simulink model "EV_Modeling"  (R2024b)
settings: Solver=FixedStepAuto  StartTime=0.0  StopTime=3500  FixedStep=0.1  RelTol=1e-3
values from neighbouring files (symbols this model uses):
  battery_SOC_resistance = battery_SOC(:,3)    [EV_Truck.m]
  battery_SOC_SOC = battery_SOC(:,1)    [EV_Truck.m]    (also in simulink.m)
  battery_SOC_voltage = battery_SOC(:,2)    [EV_Truck.m]    (also in simulink.m)
  electric_consumption_ressistancce = electric_consumption(:,2)    [EV_Truck.m]    (also in simulink.m)
  electric_consumption_voltage = electric_consumption(:,1)    [EV_Truck.m]    (also in simulink.m)
  motor_efficiency_efficiency = table2array(motor_efficiency(2:height(motor_efficiency),2:width(motor_efficiency)))    [EV_Truck.m]    (also in simulink.m)
  motor_efficiency_RPM = table2array(motor_efficiency(2:height(motor_efficiency),1))    [EV_Truck.m]    (also in simulink.m)
  motor_efficiency_torque = transpose(motor_efficiency_torque)    [EV_Truck.m]    (also in simulink.m)
  motor_RPM_torque = table2array(motor_torque(1:14,1))    [EV_Truck.m]    (also in simulink.m)
  motor_torque_RPM = table2array(motor_torque(1:14,2))    [EV_Truck.m]    (also in simulink.m)
undefined symbols (not defined in the file or in its folder): battery_builder_rtmsupport, battery_sli_rtmsupport, DiscIntNeverNeededParam, gcbh, recurrentNet
libraries: dlutilitylib x10, dlsequencelib x10, packLibrary_lib x10, simulink x7, dlconvfclib x6, dlactivationlib x5, sharedTrackingLibrary x3, mpcadaslib x2, nesl_utility x2, fl_lib x2, slpidlib x2, simulink_extras x1
(part 8 of 9)

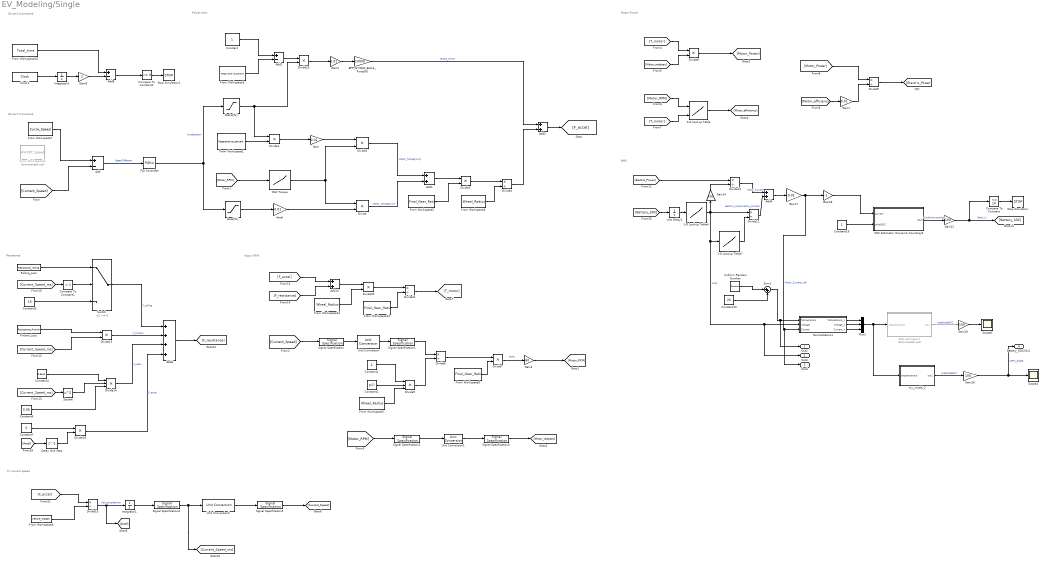
== system EV_Modeling/Single ==
  note: BMS
  note: To current speed
  note: Resistance
  note: Motor Power
  note: Power train
  note: Driver's Command
  note: RPS
  note: Motor RPM
  note: Driver's Command
  " Normalization1" : MATLAB Function  TreatAsAtomicUnit=on
  1-D Lookup Table4 : Lookup_n-D  NumberOfTableDimensions=1  BreakpointsForDimension1=battery_SOC_SOC  Table=battery_SOC_voltage  ExtrapMethod=Clip  UseLastTableValue=on  InternalRulePriority=Speed  RndMeth=Simplest
  1-D Lookup Table7 : Lookup_n-D  NumberOfTableDimensions=1  BreakpointsForDimension1=battery_SOC_SOC  Table=battery_SOC_resistance  InternalRulePriority=Speed  RndMeth=Simplest
  2-D Lookup Table : Lookup_n-D  BreakpointsForDimension1=motor_efficiency_RPM  BreakpointsForDimension2=motor_efficiency_torque  Table=motor_efficiency_efficiency  InternalRulePriority=Speed  RndMeth=Simplest
      settings: InputPortMap=u0,u1
  Accel : Gain  Gain=0.01
  Accel[%] : Saturate  UpperLimit=100  LowerLimit=0
  Add : Sum  Inputs=+-
  Add{1,3..4,10} (4 alike) : Sum
  Add2 : Sum  Inputs=+-
  Add6 : Sum  Inputs=++++
  Add8 : Sum  Inputs=+-
  BPP[%]*MAX_Brake_Force[N] : Gain  Gain=10000
  Brake[%] : Saturate  UpperLimit=0  LowerLimit=-100
  Clock1 : simulink_extras/Flip Flops/Clock  period=2
  Compare To Constant : simulink/Logic and Bit Operations/Compare To Constant  relop=<=  const=10  OutDataTypeStr=boolean
  Compare To Constant1 : simulink/Logic and Bit Operations/Compare To Constant  relop=>  const=1  OutDataTypeStr=boolean
  Compare To Constant2 : simulink/Logic and Bit Operations/Compare To Constant  relop=<=  const=0  OutDataTypeStr=boolean
  Constant : Constant
  Constant1 : Constant  Value=2
  Constant13 : Constant  Value=25
  Constant16 : Constant
  Constant2 : Constant  Value=pi()
  Constant3 : Constant  Value=10
  Constant4 : Constant  Value=0.6441
  Constant6 : Constant  Value=5.06
  Constant7 : Constant  Value=5
  Delay One Step : Delay  DelayLength=1
  Divide{,1..3,7..8,13,16,19..20} (10 alike) : Product  Inputs=**
  Divide{4,6,9,11..12,15,21} (7 alike) : Product  Inputs=*/
  Divide14 : Product  Inputs=***
  Divide5 : Product  Inputs=***
  Friction_Loss : FromWorkspace  VariableName=Resistance_friction
  From Workspace1 : FromWorkspace  VariableName=Regenerative_percent
  From Workspace10 : FromWorkspace  VariableName=Total_time
  From Workspace11 : FromWorkspace  Commented=on  VariableName=HWFET_Speed
  From Workspace12 : FromWorkspace  VariableName=Final_Gear_Ratio
  From Workspace13 : FromWorkspace  VariableName=Wheel_Radius
  From Workspace2 : FromWorkspace  VariableName=Final_Gear_Ratio
  From Workspace3 : FromWorkspace  VariableName=Regenerative_percent
  From Workspace4 : FromWorkspace  VariableName=Wheel_Radius
  From Workspace5 : FromWorkspace  VariableName=Wheel_Radius
  From Workspace6 : FromWorkspace  VariableName=Final_Gear_Ratio
  From Workspace7 : FromWorkspace  VariableName=Cycle_Speed
  From Workspace9 : FromWorkspace  VariableName=Vehicle_Weight
  Gain{,1,7,17} (4 alike) : Gain  Gain=0.01
  Gain{12,14,16,19} (4 alike) : Gain  Gain=100
  Gain18 : Gain  Gain=-1
  Gain2 : Gain  Gain=60
  Gain8 : Gain  Gain=2
  Integrator1 : Integrator
  Integrator3 : Integrator
  MAX Torque : Lookup_n-D  NumberOfTableDimensions=1  BreakpointsForDimension1=motor_RPM_torque  Table=motor_torque_RPM  InternalRulePriority=Speed  RndMeth=Simplest
  Mux2 : Mux  Inputs=3
  PID Controller : slpidlib/PID Controller  Controller=PID  Form=Parallel  TimeDomain=Continuous-time  UseExternalTs=off  SampleTime=-1  IntegratorMethod=Forward Euler  FilterMethod=Forward Euler  ControllerParametersSource=internal  P=100  I=0.01  UseKiTs=off  D=0.0001  UseExternalDerivativeSource=off  N=10  UseFilter=on  TunerSelectOption=Transfer Function Based (PID Tuner App)  InitialConditionSource=internal  InitialConditionForIntegrator=0  InitialConditionForFilter=0  DifferentiatorICPrevScaledInput=0  ExternalReset=none  TrackingMode=off  Kt=1  LimitOutput=off  SatLimitsSource=internal  UpperSaturationLimit=inf  LowerSaturationLimit=-inf  LinearizeAsGain=on  AntiWindupMode=none  Kb=1  LimitIntegrator=off  UpperIntegratorSaturationLimit=inf  LowerIntegratorSaturationLimit=-inf  POutMin=[]  POutMax=[]  IOutMin=[]  IOutMax=[]  DOutMin=[]  DOutMax=[]  NOutMin=[]  NOutMax=[]  SumOutMin=[]  SumOutMax=[]  SaturationOutMin=[]  SaturationOutMax=[]  PParamMin=[]  PParamMax=[]  IParamMin=[]  IParamMax=[]  DParamMin=[]  DParamMax=[]  NParamMin=[]  NParamMax=[]  KbParamMin=[]  KbParamMax=[]  KtParamMin=[]  KtParamMax=[]  KbOutMin=[]  KbOutMax=[]  KtOutMin=[]  KtOutMax=[]  IntegratorOutMin=[]  IntegratorOutMax=[]  FilterOutMin=[]  FilterOutMax=[]  SumI1OutMin=[]  SumI1OutMax=[]  SumI2OutMin=[]  SumI2OutMax=[]  SumI3OutMin=[]  SumI3OutMax=[]  SumI4OutMin=[]  SumI4OutMax=[]  SumDOutMin=[]  SumDOutMax=[]  DifferentiatorOutMin=[]  DifferentiatorOutMax=[]  FilterDiffOutCoefMin=[]  FilterDiffOutCoefMax=[]  ReciprocalOutMin=[]  ReciprocalOutMax=[]  SumDenOutMin=[]  SumDenOutMax=[]  SumNumOutMin=[]  SumNumOutMax=[]  DivideOutMin=[]  DivideOutMax=[]  UdiffTsProdOutMin=[]  UdiffTsProdOutMax=[]  NTsProdOutMin=[]  NTsProdOutMax=[]  UintegralTsProdOutMin=[]  UintegralTsProdOutMax=[]  UngainTsProdOutMin=[]  UngainTsProdOutMax=[]  ClampingZeroOutDataTypeStr=Inherit: Inherit via back propagation  ClampingZeroOutMin=[]  ClampingZeroOutMax=[]  FilterDenConstantOutDataTypeStr=Inherit: Inherit via back propagation  FilterDenConstantOutMin=[]  FilterDenConstantOutMax=[]  PCopyOutDataTypeStr=Inherit: Inherit via back propagation  PCopyOutMin=[]  PCopyOutMax=[]  NCopyOutDataTypeStr=Inherit: Inherit via back propagation  NCopyOutMin=[]  NCopyOutMax=[]  IntegratorContinuousStateAttributes=''  IntegratorStateMustResolveToSignalObject=off  IntegratorRTWStateStorageClass=Auto  FilterContinuousStateAttributes=''  FilterStateMustResolveToSignalObject=off  FilterRTWStateStorageClass=Auto  ParallelPVariant=InternalParameters  IdealPVariant=Disabled  IVariant=InternalParameters  DVariant=InternalParameters  IntegratorVariant=Continuous  SatVariant=Disabled  AWVariant=Passthrough  PCopyVariant=Disabled  TRVariant=Disabled  FdbkBlocksVariant=Forward  IdealPFdbkVariant=Disabled  SatFdbkVariant=Disabled  DerivativeFilterVariant=ContFilter  NVariant=InternalParameters  NCopyVariant=Disabled  FilterICVariant=InternalICsFilter  IntegratorICVariant=InternalICs  ExternalResetVariant=Disabled  TRSumVariant=Passthrough  SumFdbkVariant=Disabled  SumVariant=Sum_PID  TsampFilterVariant=InternalTs  TsampNgainVariant=Passthrough  TsampIntegralVariant=Disabled_SignalSpec  ExternalSaturationOutDataTypeStr=Inherit: Same as second input  DerivativeSourceVariant=ErrorSignal  PreIntVariant=InternalPreInt
  Rolling_Loss : FromWorkspace  VariableName=Resistance_rolling
  SOC Estimator (Coulomb Counting)2 : Subsystem  AncestorBlock=|  LoadFcn=battery_sli_rtmsupport( 'loadfcn', gcbh );  TreatAsAtomicUnit=on  mask(SOC Estimator (Coulomb Counting)){CurrentInputPartition=on, AH=4.5, Ts=-1}
      | batt_sl_lib/Estimators/SOC Estimator
      | (Coulomb Counting)
      mask prompts: CurrentInputPartition "physmod:battery:library:comments:control:BatteryEstimators:SpecifyCurrentInputAsCellCurrents_MP"; AH "physmod:battery:library:comments:control:BatteryEstimators:CellCapacityAH_MP"; Ts "physmod:battery:library:comments:control:BatteryEstimators:SampleTime1ForInherited_MP"
      mask help: physmod:battery:library:comments:control:BatteryEstimators:CoulombCounting_MD
      mask init:
      | battery.mask.initializeCoulombCounter(AH,Ts);
      | battery.mask.initializeCurrentInputPartition([gcb '/For Each'],CurrentInputPartition);
      settings: CopyFcn=battery_sli_rtmsupport( 'copyfcn', gcbh );  DeleteFcn=battery_sli_rtmsupport( 'deletefcn', gcbh );  ModelCloseFcn=battery_sli_rtmsupport( 'modelclosefcn', gcbh );  PostSaveFcn=battery_sli_rtmsupport( 'postsavefcn', gcbh );  PreCopyFcn=battery_sli_rtmsupport( 'precopyfcn', gcbh );  OpenFcn=battery_sli_rtmsupport( 'openfcn', gcbh );  CloseFcn=battery_sli_rtmsupport( 'closefcn', gcbh );  PreDeleteFcn=battery_sli_rtmsupport( 'predeletefcn', gcbh );
      settings: LibrarySourceBlock=|
      | batt_sl_lib/Estimators/SOC Estimator
      | (Coulomb Counting)
      mask Help: web(nesl_help(gcbh))
      mask TypeOptions Ts: Integrator/Ts
      mask DialogControl CurrentInputPartition Prompt: 전류 입력을 셀 전류로 지정
      mask DialogControl AH Prompt: 셀 용량, AH(A*Hr)
      mask DialogControl Ts Prompt: 샘플 시간(상속된 경우 -1)
  SOC Estimator2 : Subsystem  Commented=on  TreatAsAtomicUnit=on
  Scope4 : Scope
  Scope6 : Scope
  Signal Specification : SignalSpecification  Unit=km/hr
  Signal Specification1 : SignalSpecification  Unit=m/s
  Signal Specification2 : SignalSpecification  Unit=rpm
  Signal Specification3 : SignalSpecification  Unit=rad/s
  Signal Specification4 : SignalSpecification  Unit=m/s
  Signal Specification5 : SignalSpecification  Unit=km/hr
  Square : Math  Operator=square
  Stop Simulation : Stop
  Stop Simulation1 : Stop
  Sum1 : Sum  Inputs=|++
  Switch : Switch  Criteria=u2 ~= 0  SaturateOnIntegerOverflow=off  InputSameDT=off
  Uniform Random Number : UniformRandomNumber  Minimum=0  Maximum=20  SampleTime=0.1
  Unit Conversion : UnitConversion
  Unit Conversion1 : UnitConversion
  Unit Conversion2 : UnitConversion
  Unit Delay2 : UnitDelay  SampleTime=-1  HasFrameUpgradeWarning=on
  my_model_2 : Subsystem
  Out2 : Outport
  Out3 : Outport  Port=2
  Out4 : Outport  Port=3
  Battery_SOC[%]1 : Outport  Port=4
  wires:
  Friction_Loss/1 -> Divide13/1
  Signal Specification3/1 -> [Motor_radpsec]
  From Workspace5/1 -> Divide5/3
  Divide1/1 -> Gain/1
  [Motor_RPM] -> Signal Specification2/1
  Divide/1 -> Add1/2  "Motor_Torque[N.m]"
  Divide7/1 -> Gain2/1
  Constant3/1 -> Switch/3
  Signal Specification5/1 -> [Current_Speed]
  Brake[%]/1 -> Divide16/2, Divide1/1
  Accel/1 -> Divide/2
  Compare To Constant1/1 -> Switch/2
  Switch/1 -> Add6/1  "F_rolling"
  [Current_Speed] -> Add/2
  MAX Torque/1 -> Divide2/2, Divide/1
  From Workspace1/1 -> Divide1/2
  Divide4/1 -> Add3/2
  Constant1/1 -> Divide5/1
  Rolling_Loss/1 -> Switch/1
  [T_motor] -> Divide8/1
  From Workspace9/1 -> Divide15/2
  Divide16/1 -> Gain1/1
  From Workspace3/1 -> Add2/2
  From Workspace4/1 -> Divide4/2
  Divide14/1 -> Add6/3  "F_aero"
  Add1/1 -> Divide3/1
  Add2/1 -> Divide16/1
  Divide8/1 -> [Motor_Power]
  From Workspace10/1 -> Add8/1
  [T_motor] -> 2-D Lookup Table/2
  Signal Specification/1 -> Unit Conversion/1
  Divide6/1 -> Divide7/1
  [F_accel] -> Divide15/1
  Divide3/1 -> Divide4/1
  Add/1 -> PID Controller/1  "Speed Different"
  [Motor_RPM] -> 2-D Lookup Table/1
  [Motor_Power] -> Divide9/1
  Accel[%]/1 -> Accel/1
  Gain7/1 -> Divide9/2
  Constant/1 -> Add2/1
  [Current_Speed_ms] -> Square/1
  Divide5/1 -> Divide6/2
  [Current_Speed] -> Signal Specification/1
  2-D Lookup Table/1 -> [Motor_efficiency]
  BPP[%]*MAX_Brake_Force[N]/1 -> Add3/1  "Brake_Force"
  Clock1/1 -> Integrator3/1
  [Current_Speed_ms] -> Compare To Constant1/1
  Divide9/1 -> [Electric_Power]
  Add3/1 -> [F_accel]
  Divide15/1 -> [Accel], Integrator1/1  "Veh_acceleartion"
  Add8/1 -> Compare To Constant2/1
  [Motor_RPM] -> MAX Torque/1
  Gain8/1 -> Add8/2
  Gain2/1 -> [Motor_RPM]
  Integrator3/1 -> Gain8/1
  Unit Conversion2/1 -> Signal Specification5/1
  Unit Conversion1/1 -> Signal Specification3/1
  Constant2/1 -> Divide5/2
  PID Controller/1 -> Brake[%]/1, Accel[%]/1  "Acceleration"
  Unit Conversion/1 -> Signal Specification1/1
  [Motor_efficiency] -> Gain7/1
  Signal Specification1/1 -> Divide6/1
  Divide2/1 -> Add1/1  "Motor_Torque[N.m]"
  Compare To Constant2/1 -> Stop Simulation1/1
  [Motor_radpsec] -> Divide8/2
  Divide13/1 -> Add6/2  "F_friction"
  Gain1/1 -> BPP[%]*MAX_Brake_Force[N]/1
  From Workspace2/1 -> Divide3/2
  [Current_Speed_ms] -> Divide13/2
  From Workspace6/1 -> Divide7/2
  Integrator1/1 -> Signal Specification4/1
  Signal Specification2/1 -> Unit Conversion1/1
  Square/1 -> Divide14/2
  Gain/1 -> Divide2/1
  Constant6/1 -> Divide14/3
  [Accel] -> Delay One Step/1
  Constant7/1 -> Divide19/1
  Delay One Step/1 -> Divide19/2
  Divide19/1 -> Add6/4  "F_accel"
  Signal Specification4/1 -> [Current_Speed_ms], Unit Conversion2/1
  Constant4/1 -> Divide14/1
  Add6/1 -> [F_resistance]
  [F_accel] -> Add10/1
  [F_resistance] -> Add10/2
  Divide21/1 -> [T_motor]
  Divide20/1 -> Divide21/1
  Add10/1 -> Divide20/1
  From Workspace13/1 -> Divide20/2
  From Workspace12/1 -> Divide21/2
  From Workspace7/1 -> Add/1
  Gain17/1 -> Out4/1, " Normalization1"/3(Current), Gain18/1  "Motor_Current_cell"
  Unit Delay2/1 -> 1-D Lookup Table4/1
  Constant16/1 -> SOC Estimator (Coulomb Counting)2/2(InitialSOC)
  [Battery_SOC] -> Unit Delay2/1
  [Electric_Power] -> Divide12/1
  Gain18/1 -> SOC Estimator (Coulomb Counting)2/1(Current)
  1-D Lookup Table7/1 -> Divide11/2
  Constant13/1 -> Sum1/2
  Gain12/1 -> Compare To Constant/1, [Battery_SOC]  "Real_LV"
  Gain19/1 -> Scope6/1
  Mux2/1 -> my_model_2/1(sequenceinput), SOC Estimator2/1(sequenceinput)
  Add4/1 -> Gain17/1
  Uniform Random Number/1 -> Sum1/1
  Gain14/1 -> Divide12/2
  my_model_2/1(out1) -> Gain16/1  "predictedSOC"
  " Normalization1"/3(Current_n) -> Mux2/3
  " Normalization1"/2(Voltage_n) -> Mux2/2
  Compare To Constant/1 -> Stop Simulation/1
  Divide12/1 -> Add4/1  "Motor_Current"
  SOC Estimator2/1(out1) -> Gain19/1  "predictedSOC"
  SOC Estimator (Coulomb Counting)2/1(SOC) -> Gain12/1  "Coulomb counting"
  Sum1/1 -> Out2/1, " Normalization1"/1(Temperature)
  " Normalization1"/1(Temperature_n) -> Mux2/1
  1-D Lookup Table4/1 -> 1-D Lookup Table7/1, Out3/1, " Normalization1"/2(Voltage), Gain14/1, Divide11/1  "Vsoc"
  Divide11/1 -> Add4/2  "electric_consumption_Current"
  Gain16/1 -> Scope4/1, Battery_SOC[%]1/1  "LSTM_Single"

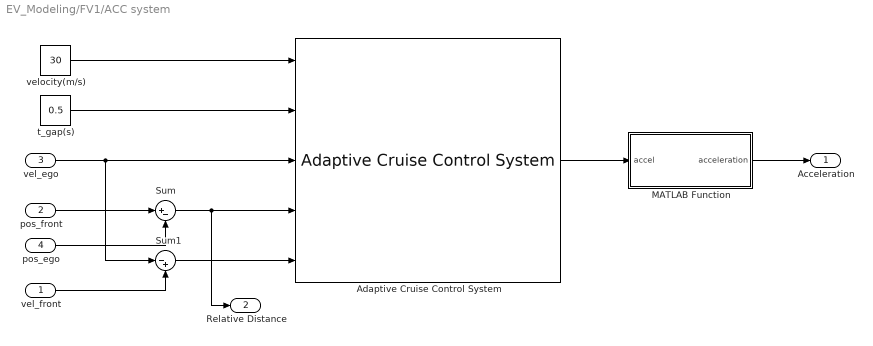
== system EV_Modeling/FV1/ACC system ==
  vel_front : Inport
  pos_front : Inport  Port=2
  vel_ego : Inport  Port=3
  pos_ego : Inport  Port=4
  Adaptive Cruise Control System : mpcadaslib/Adaptive Cruise Control System  EgoModel=tf(1,[0.5,1,0])  InitialEgoVelocity=20  DefaultSpacing=20  MaxVelocity=30  MinAcceleration=-3  amin_ext=off  MaxAcceleration=3  amax_ext=off  Ts=0.1  PredictionHorizon=100  ControllerBehavior=0.7  suboptimal=off  maxiter=10  datatypeopt=double  optmode=off  trackmode=off
      settings: LibrarySourceBlock=mpclib/Automated Driving/Adaptive Cruise Control System
  MATLAB Function : MATLAB Function  TreatAsAtomicUnit=on
  Sum : Sum  Inputs=|+-
  Sum1 : Sum  Inputs=|-+
  t_gap(s) : Constant  Value=0.5
  velocity(m/s) : Constant  Value=30
  Acceleration : Outport
  Relative Distance : Outport  Port=2
  wires:
  t_gap(s)/1 -> Adaptive Cruise Control System/2
  Sum/1 -> Relative Distance/1, Adaptive Cruise Control System/4
  Sum1/1 -> Adaptive Cruise Control System/5
  velocity(m/s)/1 -> Adaptive Cruise Control System/1
  Adaptive Cruise Control System/1 -> MATLAB Function/1(accel)
  pos_front/1 -> Sum/1
  pos_ego/1 -> Sum/2
  vel_front/1 -> Sum1/2
  vel_ego/1 -> Sum1/1, Adaptive Cruise Control System/3
  MATLAB Function/1(acceleration) -> Acceleration/1

== system EV_Modeling/FV1/Coulomb Counting ==
  Motor_Current_cell : Inport
  Constant13 : Constant
  Constant14 : Constant  Value=4.5*3600
  Discrete-Time Integrator : DiscreteIntegrator  SampleTime=-1  ICPrevOutput=DiscIntNeverNeededParam  ICPrevScaledInput=DiscIntNeverNeededParam
  Divide10 : Product  Inputs=*/
  Minus1 : Sum  Inputs=+-
  SOC_CC : Outport
  wires:
  Minus1/1 -> SOC_CC/1
  Motor_Current_cell/1 -> Discrete-Time Integrator/1
  Constant13/1 -> Minus1/1
  Divide10/1 -> Minus1/2
  Discrete-Time Integrator/1 -> Divide10/1
  Constant14/1 -> Divide10/2

== system EV_Modeling/FV1/LSTM ==
  sequenceinput : Inport  PortDimensions="[3  1]"
  dropout_1 : dlutilitylib/Dropout Layer  SampleTime=-1
  dropout_2 : dlutilitylib/Dropout Layer  SampleTime=-1
  fc : dlconvfclib/Fully Connected Layer  Layer=recurrentNet.Layers(6)  OutMin=[]  OutMax=[]  WeightsDataTypeStr=Inherit: Inherit via back propagation  WeightsMin=[]  WeightsMax=[]  BiasDataTypeStr=Inherit: Inherit via back propagation  BiasMin=[]  BiasMax=[]  MatrixMultiplyMin=[]  MatrixMultiplyMax=[]  SampleTime=-1
      settings: DataFormat=CT
  layer : dlactivationlib/Sigmoid Layer  ApproximationMethod=None  OutMin=[]  OutMax=[]  SampleTime=-1
  lstm_1 : dlsequencelib/LSTM Layer  Layer=recurrentNet.Layers(2)  Stateful=on  ApproximationMethod=None  InputWeightsDataTypeStr=Inherit: Inherit via back propagation  InputWeightsMin=[]  InputWeightsMax=[]  RecurrentWeightsDataTypeStr=Inherit: Inherit via back propagation  RecurrentWeightsMin=[]  RecurrentWeightsMax=[]  BiasDataTypeStr=Inherit: Inherit via back propagation  BiasMin=[]  BiasMax=[]  InitialCellStateDataTypeStr=Inherit: Inherit via back propagation  InitialCellStateMin=[]  InitialCellStateMax=[]  CellStateMin=[]  CellStateMax=[]  InitialHiddenStateDataTypeStr=Inherit: Inherit via back propagation  InitialHiddenStateMin=[]  InitialHiddenStateMax=[]  HiddenStateMin=[]  HiddenStateMax=[]  InputWeightsMatrixMultiplyOutMin=[]  InputWeightsMatrixMultiplyOutMax=[]  RecurrentWeightsMatrixMultiplyOutMin=[]  RecurrentWeightsMatrixMultiplyOutMax=[]  LinearGateAddOutMin=[]  LinearGateAddOutMax=[]  CellStateProductOutMin=[]  CellStateProductOutMax=[]  SampleTime=-1
      settings: DataFormat=CT
  lstm_2 : dlsequencelib/LSTM Layer  Layer=recurrentNet.Layers(4)  Stateful=on  ApproximationMethod=None  InputWeightsDataTypeStr=Inherit: Inherit via back propagation  InputWeightsMin=[]  InputWeightsMax=[]  RecurrentWeightsDataTypeStr=Inherit: Inherit via back propagation  RecurrentWeightsMin=[]  RecurrentWeightsMax=[]  BiasDataTypeStr=Inherit: Inherit via back propagation  BiasMin=[]  BiasMax=[]  InitialCellStateDataTypeStr=Inherit: Inherit via back propagation  InitialCellStateMin=[]  InitialCellStateMax=[]  CellStateMin=[]  CellStateMax=[]  InitialHiddenStateDataTypeStr=Inherit: Inherit via back propagation  InitialHiddenStateMin=[]  InitialHiddenStateMax=[]  HiddenStateMin=[]  HiddenStateMax=[]  InputWeightsMatrixMultiplyOutMin=[]  InputWeightsMatrixMultiplyOutMax=[]  RecurrentWeightsMatrixMultiplyOutMin=[]  RecurrentWeightsMatrixMultiplyOutMax=[]  LinearGateAddOutMin=[]  LinearGateAddOutMax=[]  CellStateProductOutMin=[]  CellStateProductOutMax=[]  SampleTime=-1
      settings: DataFormat=CT
  SOC : Outport
  wires:
  fc/1 -> layer/1
  lstm_1/1 -> dropout_1/1
  dropout_1/1 -> lstm_2/1
  layer/1 -> SOC/1
  sequenceinput/1 -> lstm_1/1
  dropout_2/1 -> fc/1
  lstm_2/1 -> dropout_2/1

== system EV_Modeling/FV2/ACC system ==
  vel_front : Inport
  pos_front : Inport  Port=2
  vel_ego : Inport  Port=3
  pos_ego : Inport  Port=4
  Adaptive Cruise Control System : mpcadaslib/Adaptive Cruise Control System  EgoModel=tf(1,[0.5,1,0])  InitialEgoVelocity=20  DefaultSpacing=20  MaxVelocity=30  MinAcceleration=-3  amin_ext=off  MaxAcceleration=3  amax_ext=off  Ts=0.1  PredictionHorizon=100  ControllerBehavior=0.7  suboptimal=off  maxiter=10  datatypeopt=double  optmode=off  trackmode=off
  MATLAB Function : MATLAB Function  TreatAsAtomicUnit=on
  Sum : Sum  Inputs=|+-
  Sum1 : Sum  Inputs=|-+
  t_gap(s) : Constant  Value=0.5
  velocity(m/s) : Constant  Value=30
  Acceleration : Outport
  Relative Distance : Outport  Port=2
  wires:
  t_gap(s)/1 -> Adaptive Cruise Control System/2
  Sum/1 -> Relative Distance/1, Adaptive Cruise Control System/4
  Sum1/1 -> Adaptive Cruise Control System/5
  velocity(m/s)/1 -> Adaptive Cruise Control System/1
  Adaptive Cruise Control System/1 -> MATLAB Function/1(accel)
  pos_front/1 -> Sum/1
  pos_ego/1 -> Sum/2
  vel_front/1 -> Sum1/2
  vel_ego/1 -> Sum1/1, Adaptive Cruise Control System/3
  MATLAB Function/1(acceleration) -> Acceleration/1

== system EV_Modeling/FV2/Coulomb Counting ==
  Motor_Current_cell : Inport
  Constant13 : Constant
  Constant14 : Constant  Value=4.5*3600
  Discrete-Time Integrator : DiscreteIntegrator  SampleTime=-1  ICPrevOutput=DiscIntNeverNeededParam  ICPrevScaledInput=DiscIntNeverNeededParam
  Divide10 : Product  Inputs=*/
  Minus1 : Sum  Inputs=+-
  SOC_CC : Outport
  wires:
  Minus1/1 -> SOC_CC/1
  Motor_Current_cell/1 -> Discrete-Time Integrator/1
  Constant13/1 -> Minus1/1
  Divide10/1 -> Minus1/2
  Discrete-Time Integrator/1 -> Divide10/1
  Constant14/1 -> Divide10/2

== system EV_Modeling/FV2/LSTM ==
  sequenceinput : Inport  PortDimensions="[3  1]"
  dropout_1 : dlutilitylib/Dropout Layer  SampleTime=-1
  dropout_2 : dlutilitylib/Dropout Layer  SampleTime=-1
  fc : dlconvfclib/Fully Connected Layer  Layer=recurrentNet.Layers(6)  OutMin=[]  OutMax=[]  WeightsDataTypeStr=Inherit: Inherit via back propagation  WeightsMin=[]  WeightsMax=[]  BiasDataTypeStr=Inherit: Inherit via back propagation  BiasMin=[]  BiasMax=[]  MatrixMultiplyMin=[]  MatrixMultiplyMax=[]  SampleTime=-1
      settings: DataFormat=CT
  layer : dlactivationlib/Sigmoid Layer  ApproximationMethod=None  OutMin=[]  OutMax=[]  SampleTime=-1
  lstm_1 : dlsequencelib/LSTM Layer  Layer=recurrentNet.Layers(2)  Stateful=on  ApproximationMethod=None  InputWeightsDataTypeStr=Inherit: Inherit via back propagation  InputWeightsMin=[]  InputWeightsMax=[]  RecurrentWeightsDataTypeStr=Inherit: Inherit via back propagation  RecurrentWeightsMin=[]  RecurrentWeightsMax=[]  BiasDataTypeStr=Inherit: Inherit via back propagation  BiasMin=[]  BiasMax=[]  InitialCellStateDataTypeStr=Inherit: Inherit via back propagation  InitialCellStateMin=[]  InitialCellStateMax=[]  CellStateMin=[]  CellStateMax=[]  InitialHiddenStateDataTypeStr=Inherit: Inherit via back propagation  InitialHiddenStateMin=[]  InitialHiddenStateMax=[]  HiddenStateMin=[]  HiddenStateMax=[]  InputWeightsMatrixMultiplyOutMin=[]  InputWeightsMatrixMultiplyOutMax=[]  RecurrentWeightsMatrixMultiplyOutMin=[]  RecurrentWeightsMatrixMultiplyOutMax=[]  LinearGateAddOutMin=[]  LinearGateAddOutMax=[]  CellStateProductOutMin=[]  CellStateProductOutMax=[]  SampleTime=-1
      settings: DataFormat=CT
  lstm_2 : dlsequencelib/LSTM Layer  Layer=recurrentNet.Layers(4)  Stateful=on  ApproximationMethod=None  InputWeightsDataTypeStr=Inherit: Inherit via back propagation  InputWeightsMin=[]  InputWeightsMax=[]  RecurrentWeightsDataTypeStr=Inherit: Inherit via back propagation  RecurrentWeightsMin=[]  RecurrentWeightsMax=[]  BiasDataTypeStr=Inherit: Inherit via back propagation  BiasMin=[]  BiasMax=[]  InitialCellStateDataTypeStr=Inherit: Inherit via back propagation  InitialCellStateMin=[]  InitialCellStateMax=[]  CellStateMin=[]  CellStateMax=[]  InitialHiddenStateDataTypeStr=Inherit: Inherit via back propagation  InitialHiddenStateMin=[]  InitialHiddenStateMax=[]  HiddenStateMin=[]  HiddenStateMax=[]  InputWeightsMatrixMultiplyOutMin=[]  InputWeightsMatrixMultiplyOutMax=[]  RecurrentWeightsMatrixMultiplyOutMin=[]  RecurrentWeightsMatrixMultiplyOutMax=[]  LinearGateAddOutMin=[]  LinearGateAddOutMax=[]  CellStateProductOutMin=[]  CellStateProductOutMax=[]  SampleTime=-1
      settings: DataFormat=CT
  SOC : Outport
  wires:
  fc/1 -> layer/1
  lstm_1/1 -> dropout_1/1
  dropout_1/1 -> lstm_2/1
  layer/1 -> SOC/1
  sequenceinput/1 -> lstm_1/1
  dropout_2/1 -> fc/1
  lstm_2/1 -> dropout_2/1

== system EV_Modeling/FV2/Subsystem ==
  Electrical Reference : fl_lib/Electrical/Electrical Elements/Electrical Reference
  Pack1 : Subsystem  LoadFcn=battery_builder_rtmsupport('loadfcn',gcbh);
      settings: CopyFcn=battery_builder_rtmsupport('copyfcn',gcbh);  PreCopyFcn=battery_builder_rtmsupport('precopyfcn',gcbh);  PreDeleteFcn=battery_builder_rtmsupport('predeletefcn',gcbh);  PortSchema="{\"entries\":[{\"content\":{\"sides\":[{\"content\":{\"connectorIds\":[\"LConn1\"]},\"type\":\"ConnectorPlacement.EquallySpacedRectSide\",\"uuid\":\"a0f968c7-f4a1-4fe7-9276-de5e3a67fc17\"},{\"content\":{\"connectorIds\":[\"RConn1\"],\"side\":\"RIGHT\"},\"type\":\"ConnectorPlacement.EquallySpacedRectSide\",\"uuid\":\"bfdc14cc-9562-4694-aabd-2d7624c7dcc1\"},{\"content\":{\"side\":\"TOP\"},\"type\":\"ConnectorPlacement.EquallySpacedRectSide\",\"uuid\":\"1e580e94-ac82-4f9b-aed9-c9ee78c93b5b\"},{\"content\":{\"connectorIds\":[\"Out1\",\"Out2\",\"Out3\",\"Out4\",\"Out5\",\"Out6\"],\"side\":\"BOTTOM\"},\"type\":\"ConnectorPlacement.EquallySpacedRectSide\",\"uuid\":\"8cc5ab0e-af37-461b-9e98-c03f53e87038\"}]},\"type\":\"ConnectorPlacement.EquallySpacedConnector\",\"uuid\":\"0e59dbb7-07bf-47a9-950b-b4945d865d6b\"}],\"packageUris\":[\"http://schema.mathworks.com/mf0/Connector/R2020b\"],\"version\":\"1.0\"}"
      mask Display: image('$imagefile')
  Solver Configuration : nesl_utility/Solver Configuration  PhysicalDomain=network_engine_domain  SubClassName=solver  LeftPortType=input  RightPortType=generic  Tones=[]  Harmonics=[]  SimulateNoise=off  Profile=off  UseLocalSampling=off  EnableSwitchedLinearOptims=on  FrequencyDomain=off  UseCCode=off  RelTol=0.001  AbsTol=0.001  MinStep=1e-09  ToWorkspace=off  RevertToSquareIcSolve=off  NumHomotopyIterations=100  PhasorMode=off  PhasorModeNumHarmonics=1  ConsistencySolver=NEWTON_XTOL_AFTER_FTOL  IndexReductionMethod=DerivativeReplacement  DoDC=on  ResidualTolerance=1e-09  ConsistencyTolSource=GLOBAL  ConsistencyAbsTol=0.001  ConsistencyRelTol=0.001  ConsistencyTolFactor=0.001  UseLocalSolver=on  LocalSolverChoice=NE_BACKWARD_EULER_ADVANCER  ResolveIndetEquations=on  FunctionEvalNumThread=1  LocalSolverSampleTime=0.1  DoFixedCost=off  MaxNonlinIter=3  MaxModeIter=2  ComputeImpulses=off  ImpulseIterations=2  LinearAlgebra=auto  LinearAlgebraNumThread=0  EquationFormulation=NE_TIME_EF  DelaysMemoryBudget=1024  AutomaticFiltering=on  FilteringTimeConstant=0.001  PartitionStorageMethod=AS_NEEDED  PartitionMemoryBudget=1024  PartitionMethod=ROBUST  MultibodyUseLocalSolver=off  MultibodyLocalSolverChoice=ODE1  MultibodyLocalSolverSampleTime=0.001
  Variable Resistor : fl_lib/Electrical/Electrical Elements/Variable Resistor  Rmin=0 Ohm  thermalEnable=false  thermal_mass=1 J/K  i_specify=off  i_priority=None  i=0 A  i_nominal_specify=off  i_nominal_value=1  i_nominal_unit=A  v_specify=off  v_priority=None  v=0 V  v_nominal_specify=off  v_nominal_value=1  v_nominal_unit=V  T_specify=off  T_priority=None  T=300 K  T_nominal_specify=off  T_nominal_value=1  T_nominal_unit=K
  Conn1 : PMIOPort  Side=Left
  iCell : Outport
  numCyclesCell : Outport  Port=2
  socCell : Outport  Port=3
  socParallelAssembly : Outport  Port=4
  vCell : Outport  Port=5
  vParallelAssembly : Outport  Port=6
  wires:
  Pack1/1(iCell) -> iCell/1
  Pack1/2(numCyclesCell) -> numCyclesCell/1
  Pack1/4(socParallelAssembly) -> socParallelAssembly/1
  Pack1/5(vCell) -> vCell/1
  Pack1/6(vParallelAssembly) -> vParallelAssembly/1
  Pack1/3(socCell) -> socCell/1  "socCell"
  connections:
  Pack1/RConn1 -- Electrical Reference/LConn1 -- Solver Configuration/RConn1 -- Variable Resistor/LConn2
  Conn1/RConn1 -- Variable Resistor/LConn1
  Pack1/LConn1 -- Variable Resistor/RConn1

== system EV_Modeling/LV/Coulomb Counting ==
  Motor_Current_cell : Inport
  Constant13 : Constant
  Constant14 : Constant  Value=4.5*3600
  Discrete-Time Integrator : DiscreteIntegrator  SampleTime=-1  ICPrevOutput=DiscIntNeverNeededParam  ICPrevScaledInput=DiscIntNeverNeededParam
  Divide10 : Product  Inputs=*/
  Minus1 : Sum  Inputs=+-
  SOC_CC : Outport
  wires:
  Minus1/1 -> SOC_CC/1
  Motor_Current_cell/1 -> Discrete-Time Integrator/1
  Constant13/1 -> Minus1/1
  Divide10/1 -> Minus1/2
  Discrete-Time Integrator/1 -> Divide10/1
  Constant14/1 -> Divide10/2

== system EV_Modeling/LV/LSTM ==
  sequenceinput : Inport  PortDimensions="[3  1]"
  dropout_1 : dlutilitylib/Dropout Layer  SampleTime=-1
  dropout_2 : dlutilitylib/Dropout Layer  SampleTime=-1
  fc : dlconvfclib/Fully Connected Layer  Layer=recurrentNet.Layers(6)  OutMin=[]  OutMax=[]  WeightsDataTypeStr=Inherit: Inherit via back propagation  WeightsMin=[]  WeightsMax=[]  BiasDataTypeStr=Inherit: Inherit via back propagation  BiasMin=[]  BiasMax=[]  MatrixMultiplyMin=[]  MatrixMultiplyMax=[]  SampleTime=-1
      settings: DataFormat=CT
  layer : dlactivationlib/Sigmoid Layer  ApproximationMethod=None  OutMin=[]  OutMax=[]  SampleTime=-1
  lstm_1 : dlsequencelib/LSTM Layer  Layer=recurrentNet.Layers(2)  Stateful=on  ApproximationMethod=None  InputWeightsDataTypeStr=Inherit: Inherit via back propagation  InputWeightsMin=[]  InputWeightsMax=[]  RecurrentWeightsDataTypeStr=Inherit: Inherit via back propagation  RecurrentWeightsMin=[]  RecurrentWeightsMax=[]  BiasDataTypeStr=Inherit: Inherit via back propagation  BiasMin=[]  BiasMax=[]  InitialCellStateDataTypeStr=Inherit: Inherit via back propagation  InitialCellStateMin=[]  InitialCellStateMax=[]  CellStateMin=[]  CellStateMax=[]  InitialHiddenStateDataTypeStr=Inherit: Inherit via back propagation  InitialHiddenStateMin=[]  InitialHiddenStateMax=[]  HiddenStateMin=[]  HiddenStateMax=[]  InputWeightsMatrixMultiplyOutMin=[]  InputWeightsMatrixMultiplyOutMax=[]  RecurrentWeightsMatrixMultiplyOutMin=[]  RecurrentWeightsMatrixMultiplyOutMax=[]  LinearGateAddOutMin=[]  LinearGateAddOutMax=[]  CellStateProductOutMin=[]  CellStateProductOutMax=[]  SampleTime=-1
      settings: DataFormat=CT
  lstm_2 : dlsequencelib/LSTM Layer  Layer=recurrentNet.Layers(4)  Stateful=on  ApproximationMethod=None  InputWeightsDataTypeStr=Inherit: Inherit via back propagation  InputWeightsMin=[]  InputWeightsMax=[]  RecurrentWeightsDataTypeStr=Inherit: Inherit via back propagation  RecurrentWeightsMin=[]  RecurrentWeightsMax=[]  BiasDataTypeStr=Inherit: Inherit via back propagation  BiasMin=[]  BiasMax=[]  InitialCellStateDataTypeStr=Inherit: Inherit via back propagation  InitialCellStateMin=[]  InitialCellStateMax=[]  CellStateMin=[]  CellStateMax=[]  InitialHiddenStateDataTypeStr=Inherit: Inherit via back propagation  InitialHiddenStateMin=[]  InitialHiddenStateMax=[]  HiddenStateMin=[]  HiddenStateMax=[]  InputWeightsMatrixMultiplyOutMin=[]  InputWeightsMatrixMultiplyOutMax=[]  RecurrentWeightsMatrixMultiplyOutMin=[]  RecurrentWeightsMatrixMultiplyOutMax=[]  LinearGateAddOutMin=[]  LinearGateAddOutMax=[]  CellStateProductOutMin=[]  CellStateProductOutMax=[]  SampleTime=-1
      settings: DataFormat=CT
  SOC : Outport
  wires:
  fc/1 -> layer/1
  lstm_1/1 -> dropout_1/1
  dropout_1/1 -> lstm_2/1
  layer/1 -> SOC/1
  sequenceinput/1 -> lstm_1/1
  dropout_2/1 -> fc/1
  lstm_2/1 -> dropout_2/1

== system EV_Modeling/Single/SOC Estimator (Coulomb Counting)2 ==
  Current : Inport  Partition=on  PartitionDimension=1  PartitionWidth=1  PartitionOffset=0
  InitialSOC : Inport  Port=2  Partition=on  PartitionDimension=1  PartitionWidth=1  PartitionOffset=0
  For Each : ForEach  DisableCoverage=on  IterateSubsysMaskParameter=off,off,off
  Gain : Gain  Gain=1/(AH*3600)
  Integrator : Subsystem  Variant=on  VariantControlMode=label  VariantControl=Choice  LabelModeActiveChoice=Discrete  mask{Ts=Ts}
      mask prompts: Ts "Sample time (-1 for inherited)"
      mask init:
      | battery.mask.refreshVariants(gcb,Ts);
  SOC : Outport  ConcatenationDimension=1
  wires:
  Integrator/1(y) -> SOC/1
  Gain/1 -> Integrator/1(u)
  InitialSOC/1 -> Integrator/2(x0)
  Current/1 -> Gain/1

== system EV_Modeling/Single/SOC Estimator2 ==
  sequenceinput : Inport  PortDimensions="[3  1]"
  my_model_placeholder : Subsystem
  out1 : Outport
  wires:
  my_model_placeholder/1(out1) -> out1/1
  sequenceinput/1 -> my_model_placeholder/1(sequenceinput)

== system EV_Modeling/Single/my_model_2 ==
  sequenceinput : Inport  PortDimensions="[3  1]"
  dropout_1 : dlutilitylib/Dropout Layer  SampleTime=-1
  dropout_2 : dlutilitylib/Dropout Layer  SampleTime=-1
  fc : dlconvfclib/Fully Connected Layer  Layer=recurrentNet.Layers(6)  OutMin=[]  OutMax=[]  WeightsDataTypeStr=Inherit: Inherit via back propagation  WeightsMin=[]  WeightsMax=[]  BiasDataTypeStr=Inherit: Inherit via back propagation  BiasMin=[]  BiasMax=[]  MatrixMultiplyMin=[]  MatrixMultiplyMax=[]  SampleTime=-1
      settings: DataFormat=CT
  layer : dlactivationlib/Sigmoid Layer  ApproximationMethod=None  OutMin=[]  OutMax=[]  SampleTime=-1
  lstm_1 : dlsequencelib/LSTM Layer  Layer=recurrentNet.Layers(2)  Stateful=on  ApproximationMethod=None  InputWeightsDataTypeStr=Inherit: Inherit via back propagation  InputWeightsMin=[]  InputWeightsMax=[]  RecurrentWeightsDataTypeStr=Inherit: Inherit via back propagation  RecurrentWeightsMin=[]  RecurrentWeightsMax=[]  BiasDataTypeStr=Inherit: Inherit via back propagation  BiasMin=[]  BiasMax=[]  InitialCellStateDataTypeStr=Inherit: Inherit via back propagation  InitialCellStateMin=[]  InitialCellStateMax=[]  CellStateMin=[]  CellStateMax=[]  InitialHiddenStateDataTypeStr=Inherit: Inherit via back propagation  InitialHiddenStateMin=[]  InitialHiddenStateMax=[]  HiddenStateMin=[]  HiddenStateMax=[]  InputWeightsMatrixMultiplyOutMin=[]  InputWeightsMatrixMultiplyOutMax=[]  RecurrentWeightsMatrixMultiplyOutMin=[]  RecurrentWeightsMatrixMultiplyOutMax=[]  LinearGateAddOutMin=[]  LinearGateAddOutMax=[]  CellStateProductOutMin=[]  CellStateProductOutMax=[]  SampleTime=-1
      settings: DataFormat=CT
  lstm_2 : dlsequencelib/LSTM Layer  Layer=recurrentNet.Layers(4)  Stateful=on  ApproximationMethod=None  InputWeightsDataTypeStr=Inherit: Inherit via back propagation  InputWeightsMin=[]  InputWeightsMax=[]  RecurrentWeightsDataTypeStr=Inherit: Inherit via back propagation  RecurrentWeightsMin=[]  RecurrentWeightsMax=[]  BiasDataTypeStr=Inherit: Inherit via back propagation  BiasMin=[]  BiasMax=[]  InitialCellStateDataTypeStr=Inherit: Inherit via back propagation  InitialCellStateMin=[]  InitialCellStateMax=[]  CellStateMin=[]  CellStateMax=[]  InitialHiddenStateDataTypeStr=Inherit: Inherit via back propagation  InitialHiddenStateMin=[]  InitialHiddenStateMax=[]  HiddenStateMin=[]  HiddenStateMax=[]  InputWeightsMatrixMultiplyOutMin=[]  InputWeightsMatrixMultiplyOutMax=[]  RecurrentWeightsMatrixMultiplyOutMin=[]  RecurrentWeightsMatrixMultiplyOutMax=[]  LinearGateAddOutMin=[]  LinearGateAddOutMax=[]  CellStateProductOutMin=[]  CellStateProductOutMax=[]  SampleTime=-1
      settings: DataFormat=CT
  out1 : Outport
  wires:
  fc/1 -> layer/1
  lstm_1/1 -> dropout_1/1
  dropout_1/1 -> lstm_2/1
  layer/1 -> out1/1
  sequenceinput/1 -> lstm_1/1
  dropout_2/1 -> fc/1
  lstm_2/1 -> dropout_2/1

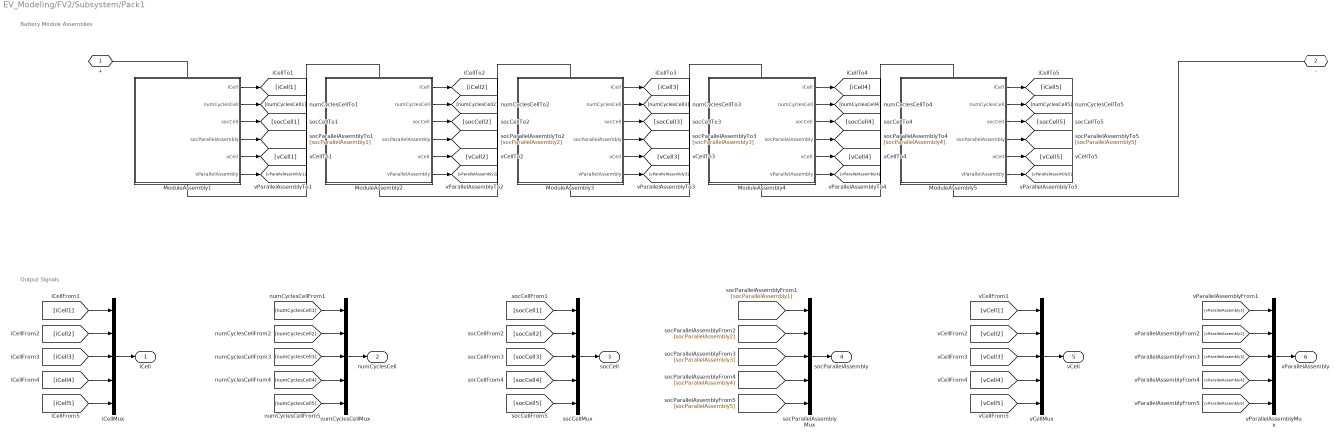
== system EV_Modeling/FV2/Subsystem/Pack1 ==
  note: Output Signals
  note: Battery Module Assemblies
  ModuleAssembly1 : Subsystem  LoadFcn=battery_builder_rtmsupport('loadfcn',gcbh);
      settings: CopyFcn=battery_builder_rtmsupport('copyfcn',gcbh);  PreCopyFcn=battery_builder_rtmsupport('precopyfcn',gcbh);  PreDeleteFcn=battery_builder_rtmsupport('predeletefcn',gcbh);  PortSchema="{\"entries\":[{\"content\":{\"sides\":[{\"content\":{\"connectorIds\":[\"LConn1\"]},\"type\":\"ConnectorPlacement.EquallySpacedRectSide\",\"uuid\":\"a0f968c7-f4a1-4fe7-9276-de5e3a67fc17\"},{\"content\":{\"connectorIds\":[\"RConn1\"],\"side\":\"RIGHT\"},\"type\":\"ConnectorPlacement.EquallySpacedRectSide\",\"uuid\":\"bfdc14cc-9562-4694-aabd-2d7624c7dcc1\"},{\"content\":{\"side\":\"TOP\"},\"type\":\"ConnectorPlacement.EquallySpacedRectSide\",\"uuid\":\"1e580e94-ac82-4f9b-aed9-c9ee78c93b5b\"},{\"content\":{\"connectorIds\":[\"Out1\",\"Out2\",\"Out3\",\"Out4\",\"Out5\",\"Out6\"],\"side\":\"BOTTOM\"},\"type\":\"ConnectorPlacement.EquallySpacedRectSide\",\"uuid\":\"a661c4db-ec60-47db-9fbc-a2faac40b68a\"}]},\"type\":\"ConnectorPlacement.EquallySpacedConnector\",\"uuid\":\"0e59dbb7-07bf-47a9-950b-b4945d865d6b\"}],\"packageUris\":[\"http://schema.mathworks.com/mf0/Connector/R2020b\"],\"version\":\"1.0\"}"
      mask Display: image('$imagefile')
  ModuleAssembly2 : Subsystem  LoadFcn=battery_builder_rtmsupport('loadfcn',gcbh);
      settings: CopyFcn=battery_builder_rtmsupport('copyfcn',gcbh);  PreCopyFcn=battery_builder_rtmsupport('precopyfcn',gcbh);  PreDeleteFcn=battery_builder_rtmsupport('predeletefcn',gcbh);  PortSchema="{\"entries\":[{\"content\":{\"sides\":[{\"content\":{\"connectorIds\":[\"LConn1\"]},\"type\":\"ConnectorPlacement.EquallySpacedRectSide\",\"uuid\":\"a0f968c7-f4a1-4fe7-9276-de5e3a67fc17\"},{\"content\":{\"connectorIds\":[\"RConn1\"],\"side\":\"RIGHT\"},\"type\":\"ConnectorPlacement.EquallySpacedRectSide\",\"uuid\":\"bfdc14cc-9562-4694-aabd-2d7624c7dcc1\"},{\"content\":{\"side\":\"TOP\"},\"type\":\"ConnectorPlacement.EquallySpacedRectSide\",\"uuid\":\"1e580e94-ac82-4f9b-aed9-c9ee78c93b5b\"},{\"content\":{\"connectorIds\":[\"Out1\",\"Out2\",\"Out3\",\"Out4\",\"Out5\",\"Out6\"],\"side\":\"BOTTOM\"},\"type\":\"ConnectorPlacement.EquallySpacedRectSide\",\"uuid\":\"a661c4db-ec60-47db-9fbc-a2faac40b68a\"}]},\"type\":\"ConnectorPlacement.EquallySpacedConnector\",\"uuid\":\"0e59dbb7-07bf-47a9-950b-b4945d865d6b\"}],\"packageUris\":[\"http://schema.mathworks.com/mf0/Connector/R2020b\"],\"version\":\"1.0\"}"
      mask Display: image('$imagefile')
  ModuleAssembly3 : Subsystem  LoadFcn=battery_builder_rtmsupport('loadfcn',gcbh);
      settings: CopyFcn=battery_builder_rtmsupport('copyfcn',gcbh);  PreCopyFcn=battery_builder_rtmsupport('precopyfcn',gcbh);  PreDeleteFcn=battery_builder_rtmsupport('predeletefcn',gcbh);  PortSchema="{\"entries\":[{\"content\":{\"sides\":[{\"content\":{\"connectorIds\":[\"LConn1\"]},\"type\":\"ConnectorPlacement.EquallySpacedRectSide\",\"uuid\":\"a0f968c7-f4a1-4fe7-9276-de5e3a67fc17\"},{\"content\":{\"connectorIds\":[\"RConn1\"],\"side\":\"RIGHT\"},\"type\":\"ConnectorPlacement.EquallySpacedRectSide\",\"uuid\":\"bfdc14cc-9562-4694-aabd-2d7624c7dcc1\"},{\"content\":{\"side\":\"TOP\"},\"type\":\"ConnectorPlacement.EquallySpacedRectSide\",\"uuid\":\"1e580e94-ac82-4f9b-aed9-c9ee78c93b5b\"},{\"content\":{\"connectorIds\":[\"Out1\",\"Out2\",\"Out3\",\"Out4\",\"Out5\",\"Out6\"],\"side\":\"BOTTOM\"},\"type\":\"ConnectorPlacement.EquallySpacedRectSide\",\"uuid\":\"a661c4db-ec60-47db-9fbc-a2faac40b68a\"}]},\"type\":\"ConnectorPlacement.EquallySpacedConnector\",\"uuid\":\"0e59dbb7-07bf-47a9-950b-b4945d865d6b\"}],\"packageUris\":[\"http://schema.mathworks.com/mf0/Connector/R2020b\"],\"version\":\"1.0\"}"
      mask Display: image('$imagefile')
  ModuleAssembly4 : Subsystem  LoadFcn=battery_builder_rtmsupport('loadfcn',gcbh);
      settings: CopyFcn=battery_builder_rtmsupport('copyfcn',gcbh);  PreCopyFcn=battery_builder_rtmsupport('precopyfcn',gcbh);  PreDeleteFcn=battery_builder_rtmsupport('predeletefcn',gcbh);  PortSchema="{\"entries\":[{\"content\":{\"sides\":[{\"content\":{\"connectorIds\":[\"LConn1\"]},\"type\":\"ConnectorPlacement.EquallySpacedRectSide\",\"uuid\":\"a0f968c7-f4a1-4fe7-9276-de5e3a67fc17\"},{\"content\":{\"connectorIds\":[\"RConn1\"],\"side\":\"RIGHT\"},\"type\":\"ConnectorPlacement.EquallySpacedRectSide\",\"uuid\":\"bfdc14cc-9562-4694-aabd-2d7624c7dcc1\"},{\"content\":{\"side\":\"TOP\"},\"type\":\"ConnectorPlacement.EquallySpacedRectSide\",\"uuid\":\"1e580e94-ac82-4f9b-aed9-c9ee78c93b5b\"},{\"content\":{\"connectorIds\":[\"Out1\",\"Out2\",\"Out3\",\"Out4\",\"Out5\",\"Out6\"],\"side\":\"BOTTOM\"},\"type\":\"ConnectorPlacement.EquallySpacedRectSide\",\"uuid\":\"a661c4db-ec60-47db-9fbc-a2faac40b68a\"}]},\"type\":\"ConnectorPlacement.EquallySpacedConnector\",\"uuid\":\"0e59dbb7-07bf-47a9-950b-b4945d865d6b\"}],\"packageUris\":[\"http://schema.mathworks.com/mf0/Connector/R2020b\"],\"version\":\"1.0\"}"
      mask Display: image('$imagefile')
  ModuleAssembly5 : Subsystem  LoadFcn=battery_builder_rtmsupport('loadfcn',gcbh);
      settings: CopyFcn=battery_builder_rtmsupport('copyfcn',gcbh);  PreCopyFcn=battery_builder_rtmsupport('precopyfcn',gcbh);  PreDeleteFcn=battery_builder_rtmsupport('predeletefcn',gcbh);  PortSchema="{\"entries\":[{\"content\":{\"sides\":[{\"content\":{\"connectorIds\":[\"LConn1\"]},\"type\":\"ConnectorPlacement.EquallySpacedRectSide\",\"uuid\":\"a0f968c7-f4a1-4fe7-9276-de5e3a67fc17\"},{\"content\":{\"connectorIds\":[\"RConn1\"],\"side\":\"RIGHT\"},\"type\":\"ConnectorPlacement.EquallySpacedRectSide\",\"uuid\":\"bfdc14cc-9562-4694-aabd-2d7624c7dcc1\"},{\"content\":{\"side\":\"TOP\"},\"type\":\"ConnectorPlacement.EquallySpacedRectSide\",\"uuid\":\"1e580e94-ac82-4f9b-aed9-c9ee78c93b5b\"},{\"content\":{\"connectorIds\":[\"Out1\",\"Out2\",\"Out3\",\"Out4\",\"Out5\",\"Out6\"],\"side\":\"BOTTOM\"},\"type\":\"ConnectorPlacement.EquallySpacedRectSide\",\"uuid\":\"a661c4db-ec60-47db-9fbc-a2faac40b68a\"}]},\"type\":\"ConnectorPlacement.EquallySpacedConnector\",\"uuid\":\"0e59dbb7-07bf-47a9-950b-b4945d865d6b\"}],\"packageUris\":[\"http://schema.mathworks.com/mf0/Connector/R2020b\"],\"version\":\"1.0\"}"
      mask Display: image('$imagefile')
  iCellMux : Mux  Inputs=5
  numCyclesCellMux : Mux  Inputs=5
  socCellMux : Mux  Inputs=5
  socParallelAssemblyMux : Mux  Inputs=5
  vCellMux : Mux  Inputs=5
  vParallelAssemblyMux : Mux  Inputs=5
  + : PMIOPort  Side=Left
  - : PMIOPort  Port=2  Side=Right
  iCell : Outport
  numCyclesCell : Outport  Port=2
  socCell : Outport  Port=3
  socParallelAssembly : Outport  Port=4
  vCell : Outport  Port=5
  vParallelAssembly : Outport  Port=6
  wires:
  [vParallelAssembly5] -> vParallelAssemblyMux/5
  ModuleAssembly5/6(vParallelAssembly) -> [vParallelAssembly5]
  [vCell5] -> vCellMux/5
  ModuleAssembly5/5(vCell) -> [vCell5]
  [socParallelAssembly5] -> socParallelAssemblyMux/5
  ModuleAssembly5/4(socParallelAssembly) -> [socParallelAssembly5]
  [socCell5] -> socCellMux/5
  ModuleAssembly5/3(socCell) -> [socCell5]
  [numCyclesCell5] -> numCyclesCellMux/5
  ModuleAssembly5/2(numCyclesCell) -> [numCyclesCell5]
  [iCell5] -> iCellMux/5
  ModuleAssembly5/1(iCell) -> [iCell5]
  [vParallelAssembly4] -> vParallelAssemblyMux/4
  ModuleAssembly4/6(vParallelAssembly) -> [vParallelAssembly4]
  [vCell4] -> vCellMux/4
  ModuleAssembly4/5(vCell) -> [vCell4]
  [socParallelAssembly4] -> socParallelAssemblyMux/4
  ModuleAssembly4/4(socParallelAssembly) -> [socParallelAssembly4]
  [socCell4] -> socCellMux/4
  ModuleAssembly4/3(socCell) -> [socCell4]
  [numCyclesCell4] -> numCyclesCellMux/4
  ModuleAssembly4/2(numCyclesCell) -> [numCyclesCell4]
  [iCell4] -> iCellMux/4
  ModuleAssembly4/1(iCell) -> [iCell4]
  [vParallelAssembly3] -> vParallelAssemblyMux/3
  ModuleAssembly3/6(vParallelAssembly) -> [vParallelAssembly3]
  [vCell3] -> vCellMux/3
  ModuleAssembly3/5(vCell) -> [vCell3]
  [socParallelAssembly3] -> socParallelAssemblyMux/3
  ModuleAssembly3/4(socParallelAssembly) -> [socParallelAssembly3]
  [socCell3] -> socCellMux/3
  ModuleAssembly3/3(socCell) -> [socCell3]
  [numCyclesCell3] -> numCyclesCellMux/3
  ModuleAssembly3/2(numCyclesCell) -> [numCyclesCell3]
  [iCell3] -> iCellMux/3
  ModuleAssembly3/1(iCell) -> [iCell3]
  [vParallelAssembly2] -> vParallelAssemblyMux/2
  ModuleAssembly2/6(vParallelAssembly) -> [vParallelAssembly2]
  [vCell2] -> vCellMux/2
  ModuleAssembly2/5(vCell) -> [vCell2]
  [socParallelAssembly2] -> socParallelAssemblyMux/2
  ModuleAssembly2/4(socParallelAssembly) -> [socParallelAssembly2]
  [socCell2] -> socCellMux/2
  ModuleAssembly2/3(socCell) -> [socCell2]
  [numCyclesCell2] -> numCyclesCellMux/2
  ModuleAssembly2/2(numCyclesCell) -> [numCyclesCell2]
  [iCell2] -> iCellMux/2
  ModuleAssembly2/1(iCell) -> [iCell2]
  [vParallelAssembly1] -> vParallelAssemblyMux/1
  vParallelAssemblyMux/1 -> vParallelAssembly/1
  ModuleAssembly1/6(vParallelAssembly) -> [vParallelAssembly1]
  [vCell1] -> vCellMux/1
  vCellMux/1 -> vCell/1
  ModuleAssembly1/5(vCell) -> [vCell1]
  [socParallelAssembly1] -> socParallelAssemblyMux/1
  socParallelAssemblyMux/1 -> socParallelAssembly/1
  ModuleAssembly1/4(socParallelAssembly) -> [socParallelAssembly1]
  [socCell1] -> socCellMux/1
  socCellMux/1 -> socCell/1
  ModuleAssembly1/3(socCell) -> [socCell1]
  [numCyclesCell1] -> numCyclesCellMux/1
  numCyclesCellMux/1 -> numCyclesCell/1
  ModuleAssembly1/2(numCyclesCell) -> [numCyclesCell1]
  [iCell1] -> iCellMux/1
  iCellMux/1 -> iCell/1
  ModuleAssembly1/1(iCell) -> [iCell1]
  connections:
  ModuleAssembly5/RConn1 -- -/RConn1
  ModuleAssembly1/LConn1 -- +/RConn1
  ModuleAssembly5/LConn1 -- ModuleAssembly4/RConn1
  ModuleAssembly4/LConn1 -- ModuleAssembly3/RConn1
  ModuleAssembly3/LConn1 -- ModuleAssembly2/RConn1
  ModuleAssembly2/LConn1 -- ModuleAssembly1/RConn1

== system EV_Modeling/Single/SOC Estimator (Coulomb Counting)2/Integrator ==
  u : Inport
  x0 : Inport  Port=2
  Continuous : Subsystem  VariantControl=Continuous
  Discrete : Subsystem  VariantControl=Discrete
  y : Outport
